simulink model "ExoskeletonControlModel"  (R2022b)
settings: Solver=ode3  StartTime=0.0  StopTime=inf  FixedStep=Ts  RelTol=1e-3
PreLoadFcn:
  | Ts_IO204 = 0.001;
  | 
  | if ~exist('Ts', 'var')
  | Ts = 0.001;
  | end
  | if ~exist('FPGA_Frequency', 'var')
  | FPGA_Frequency = 75000000;
  | end
  | 
  | ts_IO612 = 1e-3;
  | 
  | load('TargetReached.mat')
  | load('ActualPos_inc.mat')
model workspace (MAT data in the model file):
  DeltaData : timeseries (value not decoded)
  EC45_deg2incs = 2276
  EC60_deg2inc = 5461
  EC90_deg2incs = 7111
  Enc2rad_18bit = 2.3968e-05
  Enc2rad_19bit = 1.1984e-05
  Enc2rad_20bit = 5.9921e-06
  GiulioModel : robotics.RigidBodyTree (value not decoded)
  Giulio_Spheric_model : robotics.RigidBodyTree (value not decoded)
  Offset1_ticks = 571315
  Offset2_ticks = 590938.9928
  Offset3_ticks = 457912.8279
  Offset4_ticks = 482293.9763
  Offset5_ticks = 598735.9316
  Offset_M1 = 1.12645499896
  Offset_M2 = 4.02728553608
  Offset_M3 = 5.48587511336
  Offset_M4 = 2.03717511516
  Offset_M5 = 4.4996674016
  T1_Nm : object (value not decoded)
  T2_Nm : object (value not decoded)
  TBmodel : robotics.RigidBodyTree (value not decoded)
  Ts = 0.002
  Xg : object (value not decoded)
  Yg : object (value not decoded)
  Zg : object (value not decoded)
  a2 = 0.27
  change_variable = 0
  d1 = [0 0 0 0 0 0 0 0 0 0 0 0 ... (30001 elements, 30001x1)]
  d1_1 = 0.21074
  d2 = [0 0 0 0 0 0 0 0 0 0 0 0 ... (30001 elements, 30001x1)]
  d2_1 = 0.04864
  d3 = [0 0 0 0 0 0 0 0 0 0 0 0 ... (30001 elements, 30001x1)]
  d4 = [0 0 0 0 0 0 0 0 0 0 0 0 ... (30001 elements, 30001x1)]
  d5 = [0 0 0 0 0 0 0 0 0 0 0 0 ... (30001 elements, 30001x1)]
  d6 = [0 0 0 0 0 0 0 0 0 0 0 0 ... (30001 elements, 30001x1)]
  ee_x = -0.2852
  ee_y = -0.3683
  ee_z = -0.0386
  enc2rad_EC45 = 7.6699e-06
  enc2rad_EC90 = 2.3969e-05
  k1_Nm_ticks = 0.00923
  k2_Nm_ticks = 0.0257
  k3_Nm_ticks = 0.00692
  k4_Nm_ticks = 0.00729
  k5_Nm_ticks = 0.00641
  lower_lim_m1 = -330000
  lower_lim_m2 = -235302
  lower_lim_m3 = -132865
  lower_lim_m4 = -152732
  lower_lim_m5 = -138363
  lower_lim_m6 = -200325
  m1 = 2.441408578
  m2 = 3.750007
  m3 = 1.56250298
  m4 = 1.56250298
  m5 = 1.56250298
  m6 = 1.56250298
  n_oversampling = 8
  offset_sea_1 = 0.5547
  offset_sea_2 = 2.8595
  offset_sea_3 = 3.5058
  offset_sea_4 = 2.8586
  offset_sea_5 = 2.8736
  params : AKSIM (value not decoded)
  pos_th_neg = -180000
  pos_th_pos = 180000
  q1 = -1819347
  q2 = -196752
  q3 = -596465
  q4 = -556807
  q5 = -573932
  q6 = -489063
  sine = [0 0.187999937334 0.751998997352 1.69199492401 3.0079839574 4.6999608335 6.76791878442 9.21184953835 12.0317433196 15.2275888485 18.7993733417 22.7470825122 ... (12501 elements, 12501x1)]
  start : object (value not decoded)
  switch_admittance = 1
  t1 : object (value not decoded)
  t2 : object (value not decoded)
  torsionalStiffnes_M1 = 384.88
  torsionalStiffnes_M2 = 1500
  torsionalStiffnes_M3 = 901.97
  torsionalStiffnes_M4 = 950.86
  torsionalStiffnes_M5 = 930
  torsionalStiffnes_M6 = 914
  upper_lim_m1 = 340000
  upper_lim_m2 = 95467
  upper_lim_m3 = 164951
  upper_lim_m4 = 210607
  upper_lim_m5 = 252595
  upper_lim_m6 = 96694
  vel_th_neg = -100
  vel_th_pos = 100
  x = 0
undefined symbols (not defined in the file): C, DiscIntNeverNeededParam
libraries: canmsglib x285, speedgoatlib_IO614 x245, simulink x26, slrealtimeloglib x9, simulink_extras x6, robotmaniplib x6
(part 11 of 13)

== system ExoskeletonControlModel/DataProcessing/CST_trasparency/CST_control/SendPositionToEPOS2/receive_PDO3_m6 ==
  target_pos : Inport
  CAN Write : speedgoatlib_IO614/CAN/CAN Write  id=1  sampleTime=-1  portSelection=4  messageType=CAN  enaStatusPort=off  protl=IO614  ptIdx=3  isFDMod=0
  set_position : canmsglib/CAN Pack  MsgList=(none)  MsgName=CAN Msg  MsgIDType=Standard (11-bit identifier)  MsgIdentifier=hex2dec('401')  MsgLength=4  Remote=off  ApplyMinMax=off  BusOutput=off  SignalInfo={ 'target position', '0', '32', 'LE', 'signed', 'Standard', '0', '1', '0', '-Inf', 'Inf' }
      settings: DataFormat=manually specified signals
  wires:
  target_pos/1 -> set_position/1
  set_position/1 -> CAN Write/1

== system ExoskeletonControlModel/DataProcessing/CST_trasparency/SendTorqueCommand/Subsystem/receive_PDO4_m6 ==
  velocity_torque_offset : Inport
  Bus Selector : BusSelector  OutputSignals=target_velocity_m6,target_torque_m6,torque_offset_m6
  CAN Write : speedgoatlib_IO614/CAN/CAN Write  id=1  sampleTime=-1  portSelection=4  messageType=CAN  enaStatusPort=off  protl=IO614  ptIdx=3  isFDMod=0
  set_velocity : canmsglib/CAN Pack  MsgList=(none)  MsgName=CAN Msg  MsgIDType=Standard (11-bit identifier)  MsgIdentifier=hex2dec('504')  MsgLength=8  Remote=off  ApplyMinMax=off  BusOutput=off  SignalInfo={ 'target velocity', '0', '32', 'LE', 'signed', 'Standard', '0', '1', '0', '-Inf', 'Inf'; 'target_torque', '32', '16', 'LE', 'signed', 'Standard', '0', '1', '0', '-Inf', 'Inf'; 'torque_offset', '48', '16', 'LE', 'signed', 'Standard', '0', '1', '0', '-Inf', 'Inf' }
      settings: DataFormat=manually specified signals
  wires:
  Bus Selector/1 -> set_velocity/1  "<target_velocity_m6>"
  set_velocity/1 -> CAN Write/1
  velocity_torque_offset/1 -> Bus Selector/1
  Bus Selector/2 -> set_velocity/2  "<target_torque_m6>"
  Bus Selector/3 -> set_velocity/3  "<torque_offset_m6>"

== system ExoskeletonControlModel/DataProcessing/CST_trasparency/SendTorqueCommand/Subsystem1/receive_PDO4_m4 ==
  velocity_torque_offset : Inport
  Bus Selector : BusSelector  OutputSignals=target_velocity_m4,target_torque_m4,torque_offset_m4
  CAN Write : speedgoatlib_IO614/CAN/CAN Write  id=1  sampleTime=-1  portSelection=4  messageType=CAN  enaStatusPort=off  protl=IO614  ptIdx=3  isFDMod=0
  set_velocity : canmsglib/CAN Pack  MsgList=(none)  MsgName=CAN Msg  MsgIDType=Standard (11-bit identifier)  MsgIdentifier=hex2dec('502')  MsgLength=8  Remote=off  ApplyMinMax=off  BusOutput=off  SignalInfo={ 'target velocity', '0', '32', 'LE', 'signed', 'Standard', '0', '1', '0', '-Inf', 'Inf'; 'target_torque', '32', '16', 'LE', 'signed', 'Standard', '0', '1', '0', '-Inf', 'Inf'; 'torque_offset', '48', '16', 'LE', 'signed', 'Standard', '0', '1', '0', '-Inf', 'Inf' }
      settings: DataFormat=manually specified signals
  wires:
  Bus Selector/1 -> set_velocity/1  "<target_velocity_m4>"
  set_velocity/1 -> CAN Write/1
  velocity_torque_offset/1 -> Bus Selector/1
  Bus Selector/2 -> set_velocity/2  "<target_torque_m4>"
  Bus Selector/3 -> set_velocity/3  "<torque_offset_m4>"

== system ExoskeletonControlModel/DataProcessing/CST_trasparency/SendTorqueCommand/Subsystem2/receive_PDO4_m5 ==
  velocity_torque_offset : Inport
  Bus Selector : BusSelector  OutputSignals=target_velocity_m5,target_torque_m5,torque_offset_m5
  CAN Write : speedgoatlib_IO614/CAN/CAN Write  id=1  sampleTime=-1  portSelection=4  messageType=CAN  enaStatusPort=off  protl=IO614  ptIdx=3  isFDMod=0
  set_velocity : canmsglib/CAN Pack  MsgList=(none)  MsgName=CAN Msg  MsgIDType=Standard (11-bit identifier)  MsgIdentifier=hex2dec('503')  MsgLength=8  Remote=off  ApplyMinMax=off  BusOutput=off  SignalInfo={ 'target velocity', '0', '32', 'LE', 'signed', 'Standard', '0', '1', '0', '-Inf', 'Inf'; 'target_torque', '32', '16', 'LE', 'signed', 'Standard', '0', '1', '0', '-Inf', 'Inf'; 'torque_offset', '48', '16', 'LE', 'signed', 'Standard', '0', '1', '0', '-Inf', 'Inf' }
      settings: DataFormat=manually specified signals
  wires:
  Bus Selector/1 -> set_velocity/1  "<target_velocity_m5>"
  set_velocity/1 -> CAN Write/1
  velocity_torque_offset/1 -> Bus Selector/1
  Bus Selector/2 -> set_velocity/2  "<target_torque_m5>"
  Bus Selector/3 -> set_velocity/3  "<torque_offset_m5>"

== system ExoskeletonControlModel/DataProcessing/CST_trasparency/SendTorqueCommand/Subsystem3/receive_PDO4_m3 ==
  velocity_torque_offset : Inport
  Bus Selector : BusSelector  OutputSignals=target_velocity_m3,target_torque_m3,torque_offset_m3
  CAN Write : speedgoatlib_IO614/CAN/CAN Write  id=1  sampleTime=-1  portSelection=4  messageType=CAN  enaStatusPort=off  protl=IO614  ptIdx=3  isFDMod=0
  set_velocity : canmsglib/CAN Pack  MsgList=(none)  MsgName=CAN Msg  MsgIDType=Standard (11-bit identifier)  MsgIdentifier=hex2dec('501')  MsgLength=8  Remote=off  ApplyMinMax=off  BusOutput=off  SignalInfo={ 'target velocity', '0', '32', 'LE', 'signed', 'Standard', '0', '1', '0', '-Inf', 'Inf'; 'target_torque', '32', '16', 'LE', 'signed', 'Standard', '0', '1', '0', '-Inf', 'Inf'; 'torque_offset', '48', '16', 'LE', 'signed', 'Standard', '0', '1', '0', '-Inf', 'Inf' }
      settings: DataFormat=manually specified signals
  wires:
  velocity_torque_offset/1 -> Bus Selector/1
  set_velocity/1 -> CAN Write/1
  Bus Selector/1 -> set_velocity/1  "<target_velocity_m3>"
  Bus Selector/2 -> set_velocity/2  "<target_torque_m3>"
  Bus Selector/3 -> set_velocity/3  "<torque_offset_m3>"

== system ExoskeletonControlModel/DataProcessing/CST_trasparency/SendTorqueCommand/Subsystem4/receive_PDO4_m1 ==
  velocity_torque_offset : Inport
  Bus Selector : BusSelector  OutputSignals=target_velocity_m1,signal2,torque_offset_m1
  CAN Write : speedgoatlib_IO614/CAN/CAN Write  id=1  sampleTime=-1  portSelection=3  messageType=CAN  enaStatusPort=off  protl=IO614  ptIdx=2  isFDMod=0
  set_velocity : canmsglib/CAN Pack  MsgList=(none)  MsgName=CAN Msg  MsgIDType=Standard (11-bit identifier)  MsgIdentifier=hex2dec('501')  MsgLength=8  Remote=off  ApplyMinMax=off  BusOutput=off  SignalInfo={ 'target velocity', '0', '32', 'LE', 'signed', 'Standard', '0', '1', '0', '-Inf', 'Inf'; 'target_torque', '32', '16', 'LE', 'signed', 'Standard', '0', '1', '0', '-Inf', 'Inf'; 'torque_offset', '48', '16', 'LE', 'signed', 'Standard', '0', '1', '0', '-Inf', 'Inf' }
      settings: DataFormat=manually specified signals
  wires:
  velocity_torque_offset/1 -> Bus Selector/1
  set_velocity/1 -> CAN Write/1
  Bus Selector/1 -> set_velocity/1  "<target_velocity_m1>"
  Bus Selector/2 -> set_velocity/2  "<signal2>"
  Bus Selector/3 -> set_velocity/3  "<torque_offset_m1>"

== stateflow chart ExoskeletonControlModel/DataProcessing/Homing_State_Machine/Homing_m2 ==
  state HOMING
    state SLEEP
    state ST3_set_home_mode
    state ST4_shutdown
    state ST5_Switch_on_and_Enable_Operation
    state ST6_set_home_position
    state ST7_set_home_method
    state Wait1
    state wait2
    state ST12_Switch_on_and_Enable_Operation
    state ST11_shutdown1
    state ST_SET_ACC_LIMITS
    state ST_SET_SPEED_LIMITS
    state ST10_set_PPM
    state ST9_stop_homing
    state ST8_start_homing
    state wait4
    state wait3
    state ST13_send_target_pos
    state ST14_Abs_ref_start_immediatly
    state Wait
    state ST15_set_home_mode
    state ST_SET_POS_HIGH_LIMITS
    state ST_SET_POS_LOW_LIMITS
    state wait5
    state wait6
    (default) -> SLEEP : {Homing_status=0}
    ST3_set_home_mode -> ST3_set_home_mode [order 2] : [rx_mode~="Homing Mode (HMM)"]
    ST3_set_home_mode -> HOMING.ST4_shutdown [order 1] : [rx_mode=="Homing Mode (HMM)"]
    HOMING.ST4_shutdown -> ST5_Switch_on_and_Enable_Operation [order 1] : [stat=="Ready to switch on"]
    Wait1 -> ST3_set_home_mode : [rx_nmt=="Operational"]{Homing_status=1}
    SLEEP -> Wait1 : [hasChangedTo(event,1)]
    wait2 -> ST7_set_home_method : after(100,msec)
    ST6_set_home_position -> wait2
    ST_SET_POS_LOW_LIMITS -> SLEEP : {Homing_status=2}
    ST5_Switch_on_and_Enable_Operation -> ST6_set_home_position [order 1] : [stat=="Operation enabled"]
    HOMING.ST4_shutdown -> HOMING.ST4_shutdown [order 2] : [stat~="Ready to switch on"]
    ST5_Switch_on_and_Enable_Operation -> ST5_Switch_on_and_Enable_Operation [order 2] : [stat~="Operation enabled"]
    ST8_start_homing -> ST6_set_home_position [order 2] : [home_status=="Homing failed"]
    ST7_set_home_method -> ST8_start_homing
    ST11_shutdown1 -> ST11_shutdown1 [order 2] : [stat~="Ready to switch on"]
    ST12_Switch_on_and_Enable_Operation -> ST12_Switch_on_and_Enable_Operation [order 2] : [stat~="Operation enabled"]
    ST10_set_PPM -> wait4
    ST9_stop_homing -> ST9_stop_homing [order 2] : [stat~="Operation enabled"]
    ST9_stop_homing -> ST10_set_PPM [order 1] : [stat=="Operation enabled"]
    wait3 -> ST_SET_ACC_LIMITS : after(100,msec)
    ST_SET_SPEED_LIMITS -> wait3
    wait4 -> ST_SET_SPEED_LIMITS : after(100,msec)
    ST_SET_ACC_LIMITS -> ST11_shutdown1 : [rx_mode=="Profile Position Mode (PPM)"]
    ST11_shutdown1 -> ST12_Switch_on_and_Enable_Operation [order 1] : [stat=="Ready to switch on"]
    ST12_Switch_on_and_Enable_Operation -> ST13_send_target_pos [order 1] : [stat=="Operation enabled"]
    ST8_start_homing -> ST9_stop_homing [order 1] : [(home_status=="Homing attained")&&(rx_mode=="Homing Mode (HMM)")]
    ST15_set_home_mode -> ST15_set_home_mode [order 2] : [rx_mode~="Homing Mode (HMM)"]
    ST14_Abs_ref_start_immediatly -> HOMING.Wait
    HOMING.Wait -> ST15_set_home_mode : [target_pos=="Target reached"]
    ST13_send_target_pos -> ST14_Abs_ref_start_immediatly
    wait5 -> ST_SET_POS_HIGH_LIMITS : after(100,msec)
    ST15_set_home_mode -> wait5 [order 1] : [rx_mode=="Homing Mode (HMM)" ]
    wait6 -> ST_SET_POS_LOW_LIMITS : after(100,msec)
    ST_SET_POS_HIGH_LIMITS -> wait6
  state FAULT
    state Wait
    state ST4_shutdown
    state Fault_reset
    state Exit
    (default) -> FAULT.Wait
    FAULT.Wait -> Fault_reset : after(5,sec)
    FAULT.ST4_shutdown -> Exit : [stat=="Ready to switch on"]
    Fault_reset -> FAULT.ST4_shutdown
  (default) -> HOMING
  HOMING -> FAULT : [stat=="Fault reaction active" || stat=="Fault"]
  FAULT -> HOMING : [stat=="Ready to switch on"]
  data: sf_internal_action_state_placeholder_data local double size=1 =0; sf_internal_action_state_placeholder_data local double size=1 =0; sf_internal_action_state_placeholder_data local double size=1 =0; sf_internal_action_state_placeholder_data local double size=1 =0; sf_internal_action_state_placeholder_data local double size=1 =0; sf_internal_action_state_placeholder_data local double size=1 =0; sf_internal_action_state_placeholder_data local double size=1 =0; sf_internal_action_state_placeholder_data local double size=1 =0; sf_internal_action_state_placeholder_data local double size=1 =0; sf_internal_action_state_placeholder_data local double size=1 =0; sf_internal_action_state_placeholder_data local double size=1 =0; sf_internal_action_state_placeholder_data local double size=1 =0; sf_internal_action_state_placeholder_data local double size=1 =0; sf_internal_action_state_placeholder_data local double size=1 =0; sf_internal_action_state_placeholder_data local double size=1 =0; sf_internal_action_state_placeholder_data local double size=1 =0; sf_internal_action_state_placeholder_data local double size=1 =0; sf_internal_action_state_placeholder_data local double size=1 =0; sf_internal_action_state_placeholder_data local double size=1 =0; rx_nmt input; rx_mode input; stat input; home_status input; target_pos input; pos_ticks input; event input double; Homing_status output

== stateflow chart ExoskeletonControlModel/DataProcessing/Homing_State_Machine/Homing_m3 ==
  state HOMING
    state SLEEP
    state ST1_Enter_Pre_Operational
    state ST2_operational
    state ST3_set_home_mode
    state ST4_shutdown
    state ST5_Switch_on_and_Enable_Operation
    state ST6_set_home_position
    state ST7_set_home_method
    state wait2
    state ST12_Switch_on_and_Enable_Operation
    state ST11_shutdown1
    state ST_SET_ACC_LIMITS
    state ST_SET_SPEED_LIMITS
    state ST10_set_PPM
    state ST9_stop_homing
    state ST8_start_homing
    state wait4
    state wait3
    state ST13_send_target_pos
    state ST14_Abs_ref_start_immediatly
    state Wait
    state ST15_set_home_mode
    state ST_SET_POS_HIGH_LIMITS
    state ST_SET_POS_LOW_LIMITS
    state wait5
    state wait6
    (default) -> SLEEP : {Homing_status=0}
    ST2_operational -> ST2_operational [order 2] : [rx_nmt~="Operational"]
    ST3_set_home_mode -> ST3_set_home_mode [order 2] : [rx_mode~="Homing Mode (HMM)"]
    ST3_set_home_mode -> HOMING.ST4_shutdown [order 1] : [rx_mode=="Homing Mode (HMM)"]
    ST1_Enter_Pre_Operational -> ST2_operational [order 2] : [rx_nmt=="Pre-operational"]
    HOMING.ST4_shutdown -> ST5_Switch_on_and_Enable_Operation [order 1] : [stat=="Ready to switch on"]
    ST2_operational -> ST3_set_home_mode [order 1] : [rx_nmt=="Operational"]{Homing_status=1}
    wait2 -> ST7_set_home_method : after(100,msec)
    ST6_set_home_position -> wait2
    ST_SET_POS_LOW_LIMITS -> SLEEP : {Homing_status=2}
    ST5_Switch_on_and_Enable_Operation -> ST6_set_home_position [order 1] : [stat=="Operation enabled"]
    SLEEP -> ST1_Enter_Pre_Operational : [hasChangedTo(event,1)]
    HOMING.ST4_shutdown -> HOMING.ST4_shutdown [order 2] : [stat~="Ready to switch on"]
    ST5_Switch_on_and_Enable_Operation -> ST5_Switch_on_and_Enable_Operation [order 2] : [stat~="Operation enabled"]
    ST8_start_homing -> ST6_set_home_position [order 2] : [home_status=="Homing failed"]
    ST1_Enter_Pre_Operational -> ST1_Enter_Pre_Operational [order 1] : [rx_nmt~="Pre-operational"]
    ST7_set_home_method -> ST8_start_homing
    ST11_shutdown1 -> ST11_shutdown1 [order 2] : [stat~="Ready to switch on"]
    ST12_Switch_on_and_Enable_Operation -> ST12_Switch_on_and_Enable_Operation [order 2] : [stat~="Operation enabled"]
    ST10_set_PPM -> wait4
    ST9_stop_homing -> ST9_stop_homing [order 2] : [stat~="Operation enabled"]
    ST9_stop_homing -> ST10_set_PPM [order 1] : [stat=="Operation enabled"]
    wait3 -> ST_SET_ACC_LIMITS : after(100,msec)
    ST_SET_SPEED_LIMITS -> wait3
    wait4 -> ST_SET_SPEED_LIMITS : after(100,msec)
    ST_SET_ACC_LIMITS -> ST11_shutdown1 : [rx_mode=="Profile Position Mode (PPM)"]
    ST11_shutdown1 -> ST12_Switch_on_and_Enable_Operation [order 1] : [stat=="Ready to switch on"]
    ST12_Switch_on_and_Enable_Operation -> ST13_send_target_pos [order 1] : [stat=="Operation enabled"]
    ST8_start_homing -> ST9_stop_homing [order 1] : [(home_status=="Homing attained")&&(rx_mode=="Homing Mode (HMM)")]
    ST15_set_home_mode -> ST15_set_home_mode [order 2] : [rx_mode~="Homing Mode (HMM)"]
    ST14_Abs_ref_start_immediatly -> HOMING.Wait
    HOMING.Wait -> ST15_set_home_mode : [target_pos=="Target reached"]
    ST13_send_target_pos -> ST14_Abs_ref_start_immediatly
    wait5 -> ST_SET_POS_HIGH_LIMITS : after(100,msec)
    ST15_set_home_mode -> wait5 [order 1] : [rx_mode=="Homing Mode (HMM)" ]
    wait6 -> ST_SET_POS_LOW_LIMITS : after(100,msec)
    ST_SET_POS_HIGH_LIMITS -> wait6
  state FAULT
    state Wait
    state ST4_shutdown
    state Fault_reset
    state Exit
    (default) -> FAULT.Wait
    FAULT.Wait -> Fault_reset : after(5,sec)
    Fault_reset -> FAULT.ST4_shutdown
    FAULT.ST4_shutdown -> Exit : [stat=="Ready to switch on"]
  (default) -> HOMING
  HOMING -> FAULT : [stat=="Fault reaction active" || stat=="Fault"]
  FAULT -> HOMING : [stat=="Ready to switch on"]
  data: sf_internal_action_state_placeholder_data local double size=1 =0; sf_internal_action_state_placeholder_data local double size=1 =0; sf_internal_action_state_placeholder_data local double size=1 =0; sf_internal_action_state_placeholder_data local double size=1 =0; sf_internal_action_state_placeholder_data local double size=1 =0; sf_internal_action_state_placeholder_data local double size=1 =0; sf_internal_action_state_placeholder_data local double size=1 =0; sf_internal_action_state_placeholder_data local double size=1 =0; sf_internal_action_state_placeholder_data local double size=1 =0; sf_internal_action_state_placeholder_data local double size=1 =0; sf_internal_action_state_placeholder_data local double size=1 =0; sf_internal_action_state_placeholder_data local double size=1 =0; sf_internal_action_state_placeholder_data local double size=1 =0; sf_internal_action_state_placeholder_data local double size=1 =0; sf_internal_action_state_placeholder_data local double size=1 =0; sf_internal_action_state_placeholder_data local double size=1 =0; sf_internal_action_state_placeholder_data local double size=1 =0; sf_internal_action_state_placeholder_data local double size=1 =0; sf_internal_action_state_placeholder_data local double size=1 =0; sf_internal_action_state_placeholder_data local double size=1 =0; sf_internal_action_state_placeholder_data local double size=1 =0; rx_nmt input; rx_mode input; stat input; home_status input; target_pos input; pos_ticks input; event input double; Homing_status output

== matlab function ExoskeletonControlModel/DataProcessing/Homing_State_Machine/MATLAB Function1 ==
  data: stat input; y output string
function y = fcn(stat)
stat=dec2bin(stat,16);
interesting_bits=stat([6]);
value='';
if isequal(interesting_bits,'1') % not ready to switch on
    value = 'Target reached';
else
    value='Target failed';
end
y = string(value);

== matlab function ExoskeletonControlModel/DataProcessing/Homing_State_Machine/MATLAB Function3 ==
  data: nmt_state input; y output string
function y = fcn(nmt_state)
value = 'Bootup';
switch nmt_state
    case hex2dec('00')
        value = 'Bootup';
    case hex2dec('04')
        value = 'Stopped';
    case hex2dec('05')
        value = 'Operational';
    case hex2dec('7F')
        value = 'Pre-operational';
end
y = string(value);

== matlab function ExoskeletonControlModel/DataProcessing/Homing_State_Machine/MATLAB Function4 ==
  data: stat input; y output string
function y = fcn(stat)
stat=dec2bin(stat,16);
interesting_bits=stat([10 11 13:16])';
value='';
if isequal(interesting_bits','000000') % not ready to switch on
    value = 'Not ready to switch on';
elseif isequal(interesting_bits','100000')
    value = 'Switch on disabled';
elseif isequal(interesting_bits','010001')
    value = 'Ready to switch on';
elseif isequal(interesting_bits','010011')
    value = 'Switched on';
elseif isequal(interesting_bits','010111')
    value = 'Operation enabled';
elseif isequal(interesting_bits','000111')
    value = 'Quick stop active';
elseif isequal(interesting_bits','001111')
    value = 'Fault reaction active';
elseif isequal(interesting_bits','001000')
    value = 'Fault';
end
y = string(value);

== matlab function ExoskeletonControlModel/DataProcessing/Homing_State_Machine/MATLAB Function5 ==
  data: mode input; y output string
function y = fcn(mode)
value = 'Profile Position Mode (PPM)';
switch mode
    case 1
        value = 'Profile Position Mode (PPM)';
    case 3
        value = 'Profile Velocity Mode (PPM)';
    case 6
        value = 'Homing Mode (HMM)';
    case 8
        value = 'Cyclic Synchronous Position Mode (CSP)';
    case 9
        value = 'Cyclic Synchronous Velocity Mode (CSV)';
    case 10
        value = 'Cyclic Synchronous Torque Mode (CST)';
end

y = string(value);

== matlab function ExoskeletonControlModel/DataProcessing/Homing_State_Machine/MATLAB Function6 ==
  data: stat input; y output string
function y = fcn(stat)
stat=dec2bin(stat,16);
interesting_bits=stat([4]);
value='';
if isequal(interesting_bits,'1') % not ready to switch on
    value = 'Homing attained';
else
    value='Homing failed';
end
y = string(value);

== matlab function ExoskeletonControlModel/DataProcessing/Homing_State_Machine/MATLAB Function10 ==
  data: stat input; y output string
function y = fcn(stat)
stat=dec2bin(stat,16);
interesting_bits=stat([4]);
value='';
if isequal(interesting_bits,'1') % not ready to switch on
    value = 'Homing attained';
else
    value='Homing failed';
end
y = string(value);

== matlab function ExoskeletonControlModel/DataProcessing/Homing_State_Machine/MATLAB Function2 ==
  data: stat input; y output string
function y = fcn(stat)
stat=dec2bin(stat,16);
interesting_bits=stat([6]);
value='';
if isequal(interesting_bits,'1') % not ready to switch on
    value = 'Target reached';
else
    value='Target failed';
end
y = string(value);

== matlab function ExoskeletonControlModel/DataProcessing/Homing_State_Machine/MATLAB Function7 ==
  data: nmt_state input; y output string
function y = fcn(nmt_state)
value = 'Bootup';
switch nmt_state
    case hex2dec('00')
        value = 'Bootup';
    case hex2dec('04')
        value = 'Stopped';
    case hex2dec('05')
        value = 'Operational';
    case hex2dec('7F')
        value = 'Pre-operational';
end
y = string(value);

== matlab function ExoskeletonControlModel/DataProcessing/Homing_State_Machine/MATLAB Function8 ==
  data: stat input; y output string
function y = fcn(stat)
stat=dec2bin(stat,16);
interesting_bits=stat([10 11 13:16])';
value='';
if isequal(interesting_bits','000000') % not ready to switch on
    value = 'Not ready to switch on';
elseif isequal(interesting_bits','100000')
    value = 'Switch on disabled';
elseif isequal(interesting_bits','010001')
    value = 'Ready to switch on';
elseif isequal(interesting_bits','010011')
    value = 'Switched on';
elseif isequal(interesting_bits','010111')
    value = 'Operation enabled';
elseif isequal(interesting_bits','000111')
    value = 'Quick stop active';
elseif isequal(interesting_bits','001111')
    value = 'Fault reaction active';
elseif isequal(interesting_bits','001000')
    value = 'Fault';
end
y = string(value);

== matlab function ExoskeletonControlModel/DataProcessing/Homing_State_Machine/MATLAB Function9 ==
  data: mode input; y output string
function y = fcn(mode)
value = 'Profile Position Mode (PPM)';
switch mode
    case 1
        value = 'Profile Position Mode (PPM)';
    case 3
        value = 'Profile Velocity Mode (PPM)';
    case 6
        value = 'Homing Mode (HMM)';
    case 8
        value = 'Cyclic Synchronous Position Mode (CSP)';
    case 9
        value = 'Cyclic Synchronous Velocity Mode (CSV)';
    case 10
        value = 'Cyclic Synchronous Torque Mode (CST)';
end

y = string(value);

== matlab function ExoskeletonControlModel/DataProcessing/Homing_State_Machine/MATLAB Function11 ==
  data: stat input; y output string
function y = fcn(stat)
stat=dec2bin(stat,16);
interesting_bits=stat([6]);
value='';
if isequal(interesting_bits,'1') % not ready to switch on
    value = 'Target reached';
else
    value='Target failed';
end
y = string(value);

== matlab function ExoskeletonControlModel/DataProcessing/Homing_State_Machine/MATLAB Function12 ==
  data: nmt_state input; y output string
function y = fcn(nmt_state)
value = 'Bootup';
switch nmt_state
    case hex2dec('00')
        value = 'Bootup';
    case hex2dec('04')
        value = 'Stopped';
    case hex2dec('05')
        value = 'Operational';
    case hex2dec('7F')
        value = 'Pre-operational';
end
y = string(value);

== matlab function ExoskeletonControlModel/DataProcessing/Homing_State_Machine/MATLAB Function13 ==
  data: stat input; y output string
function y = fcn(stat)
stat=dec2bin(stat,16);
interesting_bits=stat([10 11 13:16])';
value='';
if isequal(interesting_bits','000000') % not ready to switch on
    value = 'Not ready to switch on';
elseif isequal(interesting_bits','100000')
    value = 'Switch on disabled';
elseif isequal(interesting_bits','010001')
    value = 'Ready to switch on';
elseif isequal(interesting_bits','010011')
    value = 'Switched on';
elseif isequal(interesting_bits','010111')
    value = 'Operation enabled';
elseif isequal(interesting_bits','000111')
    value = 'Quick stop active';
elseif isequal(interesting_bits','001111')
    value = 'Fault reaction active';
elseif isequal(interesting_bits','001000')
    value = 'Fault';
end
y = string(value);

== matlab function ExoskeletonControlModel/DataProcessing/Homing_State_Machine/MATLAB Function14 ==
  data: mode input; y output string
function y = fcn(mode)
value = 'Profile Position Mode (PPM)';
switch mode
    case 1
        value = 'Profile Position Mode (PPM)';
    case 3
        value = 'Profile Velocity Mode (PPM)';
    case 6
        value = 'Homing Mode (HMM)';
    case 8
        value = 'Cyclic Synchronous Position Mode (CSP)';
    case 9
        value = 'Cyclic Synchronous Velocity Mode (CSV)';
    case 10
        value = 'Cyclic Synchronous Torque Mode (CST)';
end

y = string(value);

== matlab function ExoskeletonControlModel/DataProcessing/Homing_State_Machine/MATLAB Function15 ==
  data: stat input; y output string
function y = fcn(stat)
stat=dec2bin(stat,16);
interesting_bits=stat([4]);
value='';
if isequal(interesting_bits,'1') % not ready to switch on
    value = 'Homing attained';
else
    value='Homing failed';
end
y = string(value);

== matlab function ExoskeletonControlModel/DataProcessing/Homing_State_Machine/MATLAB Function16 ==
  data: stat input; y output string
function y = fcn(stat)
stat=dec2bin(stat,16);
interesting_bits=stat([6]);
value='';
if isequal(interesting_bits,'1') % not ready to switch on
    value = 'Target reached';
else
    value='Target failed';
end
y = string(value);

== matlab function ExoskeletonControlModel/DataProcessing/Homing_State_Machine/MATLAB Function17 ==
  data: nmt_state input; y output string
function y = fcn(nmt_state)
value = 'Bootup';
switch nmt_state
    case hex2dec('00')
        value = 'Bootup';
    case hex2dec('04')
        value = 'Stopped';
    case hex2dec('05')
        value = 'Operational';
    case hex2dec('7F')
        value = 'Pre-operational';
end
y = string(value);

== matlab function ExoskeletonControlModel/DataProcessing/Homing_State_Machine/MATLAB Function18 ==
  data: stat input; y output string
function y = fcn(stat)
stat=dec2bin(stat,16);
interesting_bits=stat([10 11 13:16])';
value='';
if isequal(interesting_bits','000000') % not ready to switch on
    value = 'Not ready to switch on';
elseif isequal(interesting_bits','100000')
    value = 'Switch on disabled';
elseif isequal(interesting_bits','010001')
    value = 'Ready to switch on';
elseif isequal(interesting_bits','010011')
    value = 'Switched on';
elseif isequal(interesting_bits','010111')
    value = 'Operation enabled';
elseif isequal(interesting_bits','000111')
    value = 'Quick stop active';
elseif isequal(interesting_bits','001111')
    value = 'Fault reaction active';
elseif isequal(interesting_bits','001000')
    value = 'Fault';
end
y = string(value);

== matlab function ExoskeletonControlModel/DataProcessing/Homing_State_Machine/MATLAB Function19 ==
  data: mode input; y output string
function y = fcn(mode)
value = 'Profile Position Mode (PPM)';
switch mode
    case 1
        value = 'Profile Position Mode (PPM)';
    case 3
        value = 'Profile Velocity Mode (PPM)';
    case 6
        value = 'Homing Mode (HMM)';
    case 8
        value = 'Cyclic Synchronous Position Mode (CSP)';
    case 9
        value = 'Cyclic Synchronous Velocity Mode (CSV)';
    case 10
        value = 'Cyclic Synchronous Torque Mode (CST)';
end

y = string(value);

== matlab function ExoskeletonControlModel/DataProcessing/Homing_State_Machine/MATLAB Function20 ==
  data: stat input; y output string
function y = fcn(stat)
stat=dec2bin(stat,16);
interesting_bits=stat([4]);
value='';
if isequal(interesting_bits,'1') % not ready to switch on
    value = 'Homing attained';
else
    value='Homing failed';
end
y = string(value);

== matlab function ExoskeletonControlModel/DataProcessing/Homing_State_Machine/MATLAB Function21 ==
  data: stat input; y output string
function y = fcn(stat)
stat=dec2bin(stat,16);
interesting_bits=stat([6]);
value='';
if isequal(interesting_bits,'1') % not ready to switch on
    value = 'Target reached';
else
    value='Target failed';
end
y = string(value);

== matlab function ExoskeletonControlModel/DataProcessing/Homing_State_Machine/MATLAB Function22 ==
  data: nmt_state input; y output string
function y = fcn(nmt_state)
value = 'Bootup';
switch nmt_state
    case hex2dec('00')
        value = 'Bootup';
    case hex2dec('04')
        value = 'Stopped';
    case hex2dec('05')
        value = 'Operational';
    case hex2dec('7F')
        value = 'Pre-operational';
end
y = string(value);

== matlab function ExoskeletonControlModel/DataProcessing/Homing_State_Machine/MATLAB Function23 ==
  data: stat input; y output string
function y = fcn(stat)
stat=dec2bin(stat,16);
interesting_bits=stat([10 11 13:16])';
value='';
if isequal(interesting_bits','000000') % not ready to switch on
    value = 'Not ready to switch on';
elseif isequal(interesting_bits','100000')
    value = 'Switch on disabled';
elseif isequal(interesting_bits','010001')
    value = 'Ready to switch on';
elseif isequal(interesting_bits','010011')
    value = 'Switched on';
elseif isequal(interesting_bits','010111')
    value = 'Operation enabled';
elseif isequal(interesting_bits','000111')
    value = 'Quick stop active';
elseif isequal(interesting_bits','001111')
    value = 'Fault reaction active';
elseif isequal(interesting_bits','001000')
    value = 'Fault';
end
y = string(value);

== matlab function ExoskeletonControlModel/DataProcessing/Homing_State_Machine/MATLAB Function24 ==
  data: mode input; y output string
function y = fcn(mode)
value = 'Profile Position Mode (PPM)';
switch mode
    case 1
        value = 'Profile Position Mode (PPM)';
    case 3
        value = 'Profile Velocity Mode (PPM)';
    case 6
        value = 'Homing Mode (HMM)';
    case 8
        value = 'Cyclic Synchronous Position Mode (CSP)';
    case 9
        value = 'Cyclic Synchronous Velocity Mode (CSV)';
    case 10
        value = 'Cyclic Synchronous Torque Mode (CST)';
end

y = string(value);

== matlab function ExoskeletonControlModel/DataProcessing/Homing_State_Machine/MATLAB Function25 ==
  data: stat input; y output string
function y = fcn(stat)
stat=dec2bin(stat,16);
interesting_bits=stat([4]);
value='';
if isequal(interesting_bits,'1') % not ready to switch on
    value = 'Homing attained';
else
    value='Homing failed';
end
y = string(value);

== matlab function ExoskeletonControlModel/DataProcessing/Homing_State_Machine/MATLAB Function26 ==
  data: stat input; y output string
function y = fcn(stat)
stat=dec2bin(stat,16);
interesting_bits=stat([6]);
value='';
if isequal(interesting_bits,'1') % not ready to switch on
    value = 'Target reached';
else
    value='Target failed';
end
y = string(value);

== matlab function ExoskeletonControlModel/DataProcessing/Homing_State_Machine/MATLAB Function27 ==
  data: nmt_state input; y output string
function y = fcn(nmt_state)
value = 'Bootup';
switch nmt_state
    case hex2dec('00')
        value = 'Bootup';
    case hex2dec('04')
        value = 'Stopped';
    case hex2dec('05')
        value = 'Operational';
    case hex2dec('7F')
        value = 'Pre-operational';
end
y = string(value);

== matlab function ExoskeletonControlModel/DataProcessing/Homing_State_Machine/MATLAB Function28 ==
  data: stat input; y output string
function y = fcn(stat)
stat=dec2bin(stat,16);
interesting_bits=stat([10 11 13:16])';
value='';
if isequal(interesting_bits','000000') % not ready to switch on
    value = 'Not ready to switch on';
elseif isequal(interesting_bits','100000')
    value = 'Switch on disabled';
elseif isequal(interesting_bits','010001')
    value = 'Ready to switch on';
elseif isequal(interesting_bits','010011')
    value = 'Switched on';
elseif isequal(interesting_bits','010111')
    value = 'Operation enabled';
elseif isequal(interesting_bits','000111')
    value = 'Quick stop active';
elseif isequal(interesting_bits','001111')
    value = 'Fault reaction active';
elseif isequal(interesting_bits','001000')
    value = 'Fault';
end
y = string(value);

== matlab function ExoskeletonControlModel/DataProcessing/Homing_State_Machine/MATLAB Function29 ==
  data: mode input; y output string
function y = fcn(mode)
value = 'Profile Position Mode (PPM)';
switch mode
    case 1
        value = 'Profile Position Mode (PPM)';
    case 3
        value = 'Profile Velocity Mode (PPM)';
    case 6
        value = 'Homing Mode (HMM)';
    case 8
        value = 'Cyclic Synchronous Position Mode (CSP)';
    case 9
        value = 'Cyclic Synchronous Velocity Mode (CSV)';
    case 10
        value = 'Cyclic Synchronous Torque Mode (CST)';
end

y = string(value);

== matlab function ExoskeletonControlModel/DataProcessing/Homing_State_Machine/MATLAB Function30 ==
  data: stat input; y output string
function y = fcn(stat)
stat=dec2bin(stat,16);
interesting_bits=stat([4]);
value='';
if isequal(interesting_bits,'1') % not ready to switch on
    value = 'Homing attained';
else
    value='Homing failed';
end
y = string(value);

== stateflow chart ExoskeletonControlModel/DataProcessing/CST_trasparency/CST_control/MOTOR5/impedance_values_safe_zones2 ==
  state SafeZone_low
    state active
      y=1
      dx1=(theta-theta_low)/2276;
      new_target_torque=-k1*dx1-beta*speed
    state hard
      y=2
      dx2=(theta-theta_low_hard)/2276
      dx1=(theta-theta_low)/2276
      new_target_torque=-k1*dx1-5*k2*dx2-beta*speed;
    (default) -> SafeZone_low.active
    SafeZone_low.active -> SafeZone_low.hard : [theta < theta_low_hard]
    SafeZone_low.hard -> SafeZone_low.active : [theta >= theta_low_hard]
  state SafeZone_high
    state active
      y=5
      dx1=(theta-theta_high)/2276
      new_target_torque=-k1*dx1-beta*speed
    state hard
      y=6
      dx2=(theta-theta_high_hard)/2276
      dx1=(theta-theta_high)/2276
      new_target_torque=-k1*dx1-5*k2*dx2-beta*speed;
    (default) -> SafeZone_high.active
    SafeZone_high.active -> SafeZone_high.hard : [theta > theta_high_hard]
    SafeZone_high.hard -> SafeZone_high.active : [theta <= theta_high_hard]
  state Transparency
    en:
    k1=0.1
    k2=2
    beta=0.05
    ZH_tau_max=1
    ZL_tau_max=1
    du:
    y = 0
    new_target_torque=0
  (default) -> Transparency
  Transparency -> SafeZone_low [order 1] : [theta < theta_low]
  Transparency -> SafeZone_high [order 2] : [theta > theta_high]
  SafeZone_high -> Transparency : [theta <= theta_high && (torque< ZH_tau_max) ]
  SafeZone_low -> Transparency : [theta >= theta_low && (torque< ZL_tau_max)]
  data: theta_low_hard constant double =-142915+2276*6; theta_low constant double =-142915+2276*9; torque input; theta_high_hard constant double =257147-2276*6; theta_high constant double =257147-2276*9; theta input; speed input; new_target_torque output; dx1 local; dx2 local; y output; beta local; ZH_tau_max local; ZL_tau_max local; k1 local; k2 local
